simulink model "week3_problem1"  (R2020b)
settings: Solver=VariableStepAuto  StartTime=0.0  StopTime=10  RelTol=1e-3
settings Model: Creator=gokul  LastModifiedBy=gokul

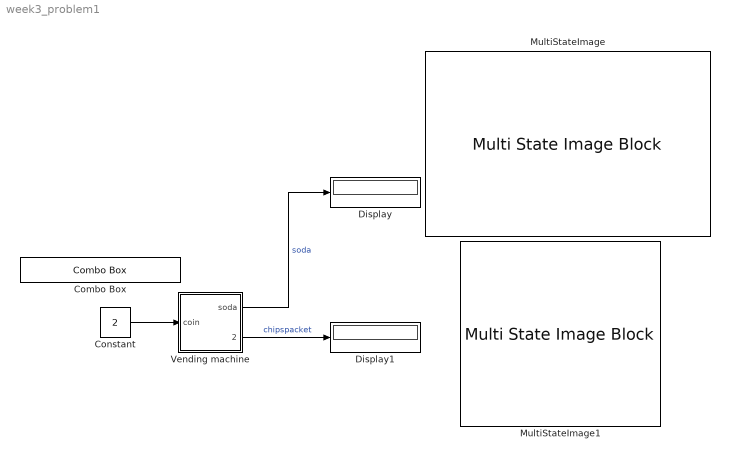
== system week3_problem1 ==
  Combo Box : ComboBox  LabelPosition=Hide  SelectedLabel=Insert two coin for soda
      settings: Values={{'No coin', 'Insert one coin for chipspacket', 'Insert two coin for soda'}, [0 1 2]}
  Constant : Constant  Value=2
  Display : Display
  Display1 : Display
  MultiStateImage : MultiStateImageBlock
  MultiStateImage1 : MultiStateImageBlock
  Vending machine : Stateflow chart  TreatAsAtomicUnit=on
  wires:
  Constant/1 -> Vending machine/1(coin)
  Vending machine/1(soda) -> Display/1  "soda"
  Vending machine/2(chipspacket) -> Display1/1  "chipspacket"

== stateflow chart week3_problem1/Vending machine ==
  state got_0
  state got_nickel
  state got_dime
  (default) -> got_0
  got_0 -> got_nickel [order 1] : [coin==1]{soda=0;chipspacket=1;}
  got_nickel -> got_0 [order 2] : [coin==2]{soda=1}
  got_dime -> got_0 [order 1] : [coin==1]{soda=1;chipspacket=1;}
  got_0 -> got_dime [order 2] : [coin==2]{soda=0;}
  got_nickel -> got_dime [order 1] : [coin==1]{soda=0;chipspacket=1;}
  got_dime -> got_nickel [order 2] : [coin==2]{soda=1;}
  data: coin input; soda output; chipspacket output
